simulink model "Ex6_IMU_SensorCharacterization"  (R2025b)
settings: Solver=FixedStepAuto  StartTime=0.0  StopTime=1800  RelTol=1e-3  EnableMultiTasking=on
libraries: simulink x7, raspberrypiCommlib x5
settings Model: ExtModeTrigDuration=2  Creator=resjoehr  LastModifiedBy=resjoehr
settings SolverCC: PositivePriorityOrder=on  AutoInsertRateTranBlk=on
settings OptimizationCC: DefaultParameterBehavior=Inlined  EnhancedBackFolding=on  PassReuseOutputArgsAs=Individual arguments  ZeroExternalMemoryAtStartup=off  ZeroInternalMemoryAtStartup=off  MaxStackSize=200000  OptimizeBlockOrder=speed  DifferentSizesBufferReuse=on  OptimizationCustomize=off  EfficientTunableParamExpr=on
settings DebuggingCC: ParameterTunabilityLossMsg=error
settings HardwareCC: ProdBitPerPointer=32.0  ProdBitPerSizeT=32.0  ProdBitPerPtrDiffT=32.0  ProdLargestAtomicInteger=Long  ProdLargestAtomicFloat=Double  ProdWordSize=32.0  ProdLongLongMode=on  ProdHWDeviceType=ARM Compatible->ARM Cortex-A (32-bit)
settings RTWCC: SystemTargetFile=ert.tlc  HardwareBoard=Raspberry Pi  TLCOptions="-aInlineSetEventsForThisBaseRateFcn=TLC_FALSE -aSuppressMultiTaskScheduler=TLC_FALSE  -aRateBasedStepFcn=0"  TemplateMakefile=ert_default_tmf  Toolchain=GNU GCC Embedded Linux  BuildConfiguration=Faster Runs  Description=Embedded Coder
settings CodeAppCC: ForceParamTrailComments=on  IgnoreCustomStorageClasses=off  OperatorAnnotations=on  SimulinkDataObjDesc=on  SFDataObjDesc=on  InsertBlockDesc=on
settings ERTTargetCC: ExtModeTransport=2.0  ExtModeStaticAlloc=on  ExtModeMexFile=ext_xcp  ExtModeIntrfLevel=Level2 - Open  CodeReplacementLibrary=ARM Cortex-A CMSIS  SupportContinuousTime=on  SupportVariableSizeSignals=on

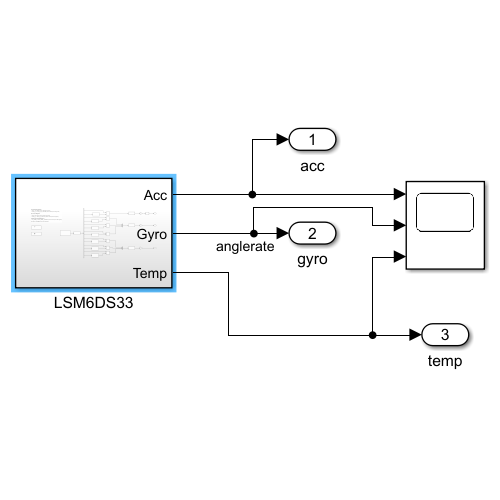
[thumbnail: Simulink's stored preview of the top-level diagram]
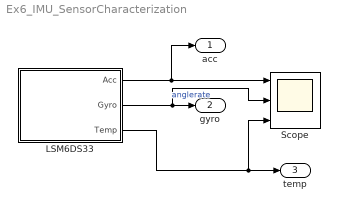
== system Ex6_IMU_SensorCharacterization ==
  LSM6DS33 : Subsystem
  Scope : Scope  NumInputPorts=3
      settings: ActiveDisplayYMinimum=-1.14514  ActiveDisplayYMaximum=0.17166
  acc : Outport
  gyro : Outport  Port=2
  temp : Outport  Port=3
  wires:
  LSM6DS33/2(Gyro) -> Scope/2, gyro/1  "anglerate"
  LSM6DS33/1(Acc) -> Scope/1, acc/1
  LSM6DS33/3(Temp) -> temp/1, Scope/3

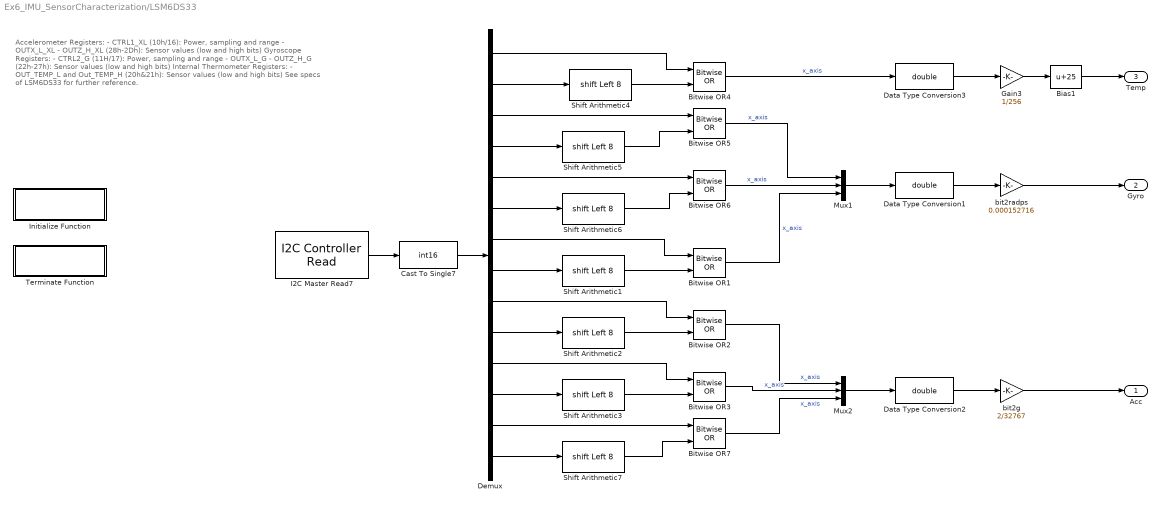
== system Ex6_IMU_SensorCharacterization/LSM6DS33 ==
  note: Accelerometer Registers:
      | - CTRL1_XL (10h/16): Power, sampling and range
      | - OUTX_L_XL - OUTZ_H_XL (28h-2Dh): Sensor values (low and high bits)
      |
      | Gyroscope Registers:
      | - CTRL2_G (11H/17): Power, sampling and range
      | - OUTX_L_G - OUTZ_H_G (22h-27h): Sensor values (low and high bits)
      |
      | Internal Thermometer Registers:
      | - OUT_TEMP_L and Out_TEMP_H (20h&21h): Sensor values (low and high bits)
      |
      | See specs of LSM6DS33 for further reference.
  Bias1 : Bias  Bias=25  SaturateOnIntegerOverflow=off
  Bitwise OR{1..7} (7 alike) : simulink/Logic and Bit Operations/Bitwise Operator  logicop=OR  UseBitMask=off  NumInputPorts=2  BitMask=bin2dec('11011001')  BitMaskRealWorld=Stored Integer
  Cast To Single7 : DataTypeConversion  OutDataTypeStr=int16  SaturateOnIntegerOverflow=off  RndMeth=Floor
  Data Type Conversion1 : DataTypeConversion  OutDataTypeStr=double  SaturateOnIntegerOverflow=off  RndMeth=Floor
  Data Type Conversion2 : DataTypeConversion  OutDataTypeStr=double  SaturateOnIntegerOverflow=off  RndMeth=Floor
  Data Type Conversion3 : DataTypeConversion  OutDataTypeStr=double  SaturateOnIntegerOverflow=off  RndMeth=Floor
  Demux : Demux  Outputs=14
  Gain3 : Gain  Gain=1/256
  I2C Master Read7 : raspberrypiCommlib/I2C Controller Read  BoardProperty=Pi 3 Model B+  I2CModule=1  Mode=Master  SlaveAddress=107  SlaveByteOrder=BigEndian  Direction=Receiver  RegisterAddressMode=on  RegisterAddress=hex2dec('20')  SlaveDataType=uint8  DataLength=14  NoAck=off  RepeatedStart=off  OutputStatus=off  SampleTime=0.01
  Initialize Function : Subsystem  TreatAsAtomicUnit=on
  Mux1 : Mux  Inputs=3
  Mux2 : Mux  Inputs=3
  Shift Arithmetic{1..7} (7 alike) : ArithShift  BitShiftNumber=8  BitShiftDirection=Left
  Terminate Function : Subsystem  TreatAsAtomicUnit=on
  bit2g : Gain  Gain=2/32767
  bit2radps : Gain  Gain=0.000152716
  Acc : Outport  Unit=g
  Gyro : Outport  Port=2  Unit=rad/s
  Temp : Outport  Port=3
  wires:
  Cast To Single7/1 -> Demux/1
  Shift Arithmetic4/1 -> Bitwise OR4/2
  Bitwise OR4/1 -> Data Type Conversion3/1  "x_axis"
  Shift Arithmetic6/1 -> Bitwise OR6/2
  Demux/1 -> Bitwise OR4/1
  Mux1/1 -> Data Type Conversion1/1
  Demux/5 -> Bitwise OR6/1
  Demux/6 -> Shift Arithmetic6/1
  I2C Master Read7/1 -> Cast To Single7/1
  Bitwise OR6/1 -> Mux1/2  "x_axis"
  Demux/4 -> Shift Arithmetic5/1
  Shift Arithmetic5/1 -> Bitwise OR5/2
  Demux/3 -> Bitwise OR5/1
  Demux/2 -> Shift Arithmetic4/1
  Bitwise OR5/1 -> Mux1/1  "x_axis"
  Data Type Conversion1/1 -> bit2radps/1
  Shift Arithmetic3/1 -> Bitwise OR3/2
  Bitwise OR3/1 -> Mux2/2  "x_axis"
  Bitwise OR1/1 -> Mux1/3  "x_axis"
  Shift Arithmetic1/1 -> Bitwise OR1/2
  Demux/7 -> Bitwise OR1/1
  Mux2/1 -> Data Type Conversion2/1
  Bitwise OR2/1 -> Mux2/1  "x_axis"
  Shift Arithmetic2/1 -> Bitwise OR2/2
  Demux/9 -> Bitwise OR2/1
  Demux/10 -> Shift Arithmetic2/1
  Demux/8 -> Shift Arithmetic1/1
  Demux/11 -> Bitwise OR3/1
  Demux/12 -> Shift Arithmetic3/1
  Demux/13 -> Bitwise OR7/1
  Shift Arithmetic7/1 -> Bitwise OR7/2
  Demux/14 -> Shift Arithmetic7/1
  Bitwise OR7/1 -> Mux2/3  "x_axis"
  Data Type Conversion2/1 -> bit2g/1
  Gain3/1 -> Bias1/1
  Bias1/1 -> Temp/1
  Data Type Conversion3/1 -> Gain3/1
  bit2g/1 -> Acc/1
  bit2radps/1 -> Gyro/1

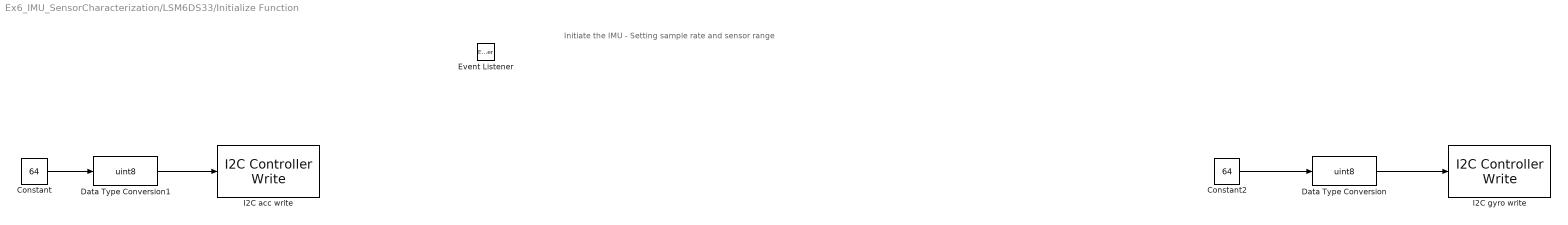
== system Ex6_IMU_SensorCharacterization/LSM6DS33/Initialize Function ==
  note: Initiate the IMU - Setting sample rate and sensor range
  Constant : Constant  Value=64
  Constant2 : Constant  Value=64
  Data Type Conversion : DataTypeConversion  OutDataTypeStr=uint8  SaturateOnIntegerOverflow=off  RndMeth=Floor
  Data Type Conversion1 : DataTypeConversion  OutDataTypeStr=uint8  SaturateOnIntegerOverflow=off  RndMeth=Floor
  Event Listener : EventListener  DisableCoverage=on  EventName=reset
  I2C acc write : raspberrypiCommlib/I2C Controller Write  BoardProperty=Pi 3 Model B+  I2CModule=1  Mode=Master  SlaveAddress=107  SlaveByteOrder=BigEndian  Direction=Transmitter  RegisterAddressMode=on  RegisterAddress=16  SlaveDataType=uint8  DataLength=1  NoAck=off  RepeatedStart=off  OutputStatus=off
  I2C gyro write : raspberrypiCommlib/I2C Controller Write  BoardProperty=Pi 3 Model B+  I2CModule=1  Mode=Master  SlaveAddress=107  SlaveByteOrder=BigEndian  Direction=Transmitter  RegisterAddressMode=on  RegisterAddress=17  SlaveDataType=uint8  DataLength=1  NoAck=off  RepeatedStart=off  OutputStatus=off
  wires:
  Constant2/1 -> Data Type Conversion/1
  Data Type Conversion/1 -> I2C gyro write/1
  Data Type Conversion1/1 -> I2C acc write/1
  Constant/1 -> Data Type Conversion1/1

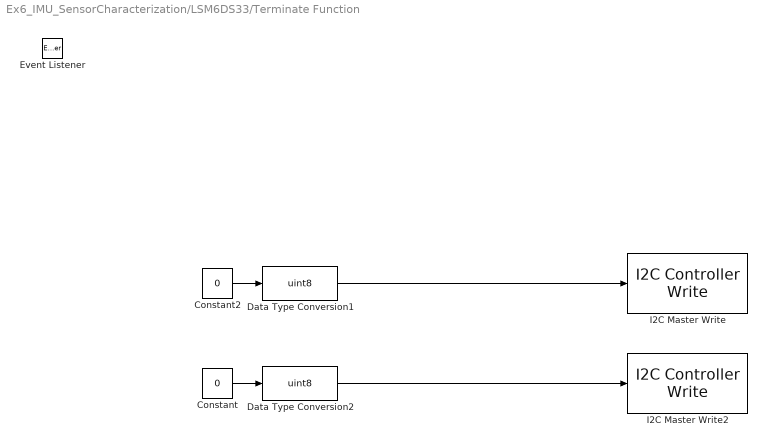
== system Ex6_IMU_SensorCharacterization/LSM6DS33/Terminate Function ==
  Constant : Constant  Value=0
  Constant2 : Constant  Value=0
  Data Type Conversion1 : DataTypeConversion  OutDataTypeStr=uint8  SaturateOnIntegerOverflow=off  RndMeth=Floor
  Data Type Conversion2 : DataTypeConversion  OutDataTypeStr=uint8  SaturateOnIntegerOverflow=off  RndMeth=Floor
  Event Listener : EventListener  DisableCoverage=on  EventType=Terminate  EventName=reset
  I2C Master Write : raspberrypiCommlib/I2C Controller Write  BoardProperty=Pi 3 Model B+  I2CModule=1  Mode=Master  SlaveAddress=107  SlaveByteOrder=BigEndian  Direction=Transmitter  RegisterAddressMode=on  RegisterAddress=17  SlaveDataType=uint8  DataLength=1  NoAck=off  RepeatedStart=off  OutputStatus=off
  I2C Master Write2 : raspberrypiCommlib/I2C Controller Write  BoardProperty=Pi 3 Model B+  I2CModule=1  Mode=Master  SlaveAddress=107  SlaveByteOrder=BigEndian  Direction=Transmitter  RegisterAddressMode=on  RegisterAddress=16  SlaveDataType=uint8  DataLength=1  NoAck=off  RepeatedStart=off  OutputStatus=off
  wires:
  Data Type Conversion1/1 -> I2C Master Write/1
  Constant/1 -> Data Type Conversion2/1
  Data Type Conversion2/1 -> I2C Master Write2/1
  Constant2/1 -> Data Type Conversion1/1
